simulink model "x5Fish_Run6"  (R2024a)
settings: Solver=VariableStepAuto  StartTime=0.0  StopTime=sim_time  FixedStep=0.0001  RelTol=1e-3
values from neighbouring files (symbols this model uses):
  A = zeros(numSets, 1)    [CurveFitting_Run4.m]    (also in MidlingFish_Run1.m = [A(1:index-1,:);A(index+1:num_search,:)]; MidliningFishOldSkelFunction.m = [A(1:index-1,:);A(index+1:num_search,:)]; calculateSegmentErrors.m = -v1(2))
  B = zeros(numSets, 1)    [CurveFitting_Run4.m]    (also in calculateSegmentErrors.m = v1(1))
  bodlen = fishlen-head    [FishSimParametersFile_Run5.m]
  bsi = NumOfSegs-1    (= 4)    [FishSimParametersFile_Run5.m]
  C = zeros(numSets, 1)    [CurveFitting_Run4.m]    (also in calculateSegmentErrors.m = -(A * startSegment(1) + B * startSegment(2)))
  D = zeros(NumOfSegs)    [FishSimParametersFile_Run5.m]
  Fish_Gain = -[1,1,1,1,1,1,1,1,1,1, 1,  1, 1, 1, 1, 1, 1, 1, 1, 1, 1, 1, 1, 1, 1, 1, 1, 1, 1, 1]    [FishSimParametersFile_Run5.m]
  fish_model_from_head = 59.1375    [FishSimParametersFile_Run5.m]
  head = fishlen*headsize_factor    [FishSimParametersFile_Run5.m]
  head_dense = head_dense*re_ratio    [DensityFinder.m]    (also in FishSimParametersFile_Run5.m = 0.76522755475)
  seglen = bodlen/bsi    [FishSimParametersFile_Run5.m]
  sim_time = t_diff*numel(midlineFiles)    [FishSimParametersFile_Run5.m]
  trunk_dense = trunk_dense*re_ratio    [DensityFinder.m]    (also in FishSimParametersFile_Run5.m = 0.76522755475)
  var_a = fish_width_half_trunk*2*lsf    (= 30.2916666667)    [FishSimParametersFile_Run5.m]
  var_b = var_a- (fish_cross_area_trunk)*(lsf^2)/var_c    (= 6.50064730042)    [FishSimParametersFile_Run5.m]
  var_c = fish_height_half*2*lsf    (= 40.8426966292)    [FishSimParametersFile_Run5.m]
undefined symbols (not defined in the file or in its folder): X, Y, Z
libraries: nesl_utility x63, sm_lib x51
(part 3 of 3)

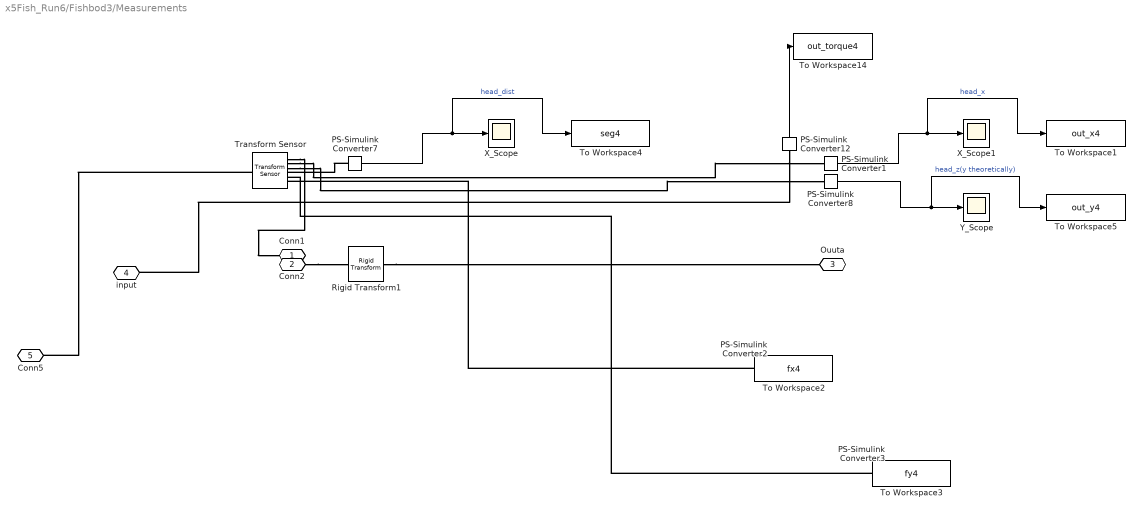
== system x5Fish_Run6/Fishbod3/Measurements ==
  PS-Simulink Converter{1..3,7..8,12} (6 alike) : nesl_utility/PS-Simulink Converter  PhysicalDomain=network_engine_domain  SubClassName=ps_output  LeftPortType=input  RightPortType=output  PseudoPeriodic=off  Frequencies=[]  VectorFormat=inherit  Unit=inherit  AffineConversion=off
  Rigid Transform1 : sm_lib/Frames and Transforms/Rigid Transform  RotationMethod=AlignedAxes  FollAlignAxisA=+Y  BaseAlignAxisA=+Z  FollAlignAxisB=+Z  BaseAlignAxisB=+Y  RotationStandardAxis=+X  RotationAngle=15  RotationAngleUnits=deg  RotationArbitraryAxis=[0 0 1]  RotationSequenceAxes=FollowerAxes  RotationSequence=XYX  RotationSequenceAngles=[0 0 0]  RotationSequenceAnglesUnits=deg  RotationMatrix=[1 0 0; 0 1 0; 0 0 1]  Quaternion=[1 0 0 0]  TranslationMethod=Cartesian  TranslationCartesianOffset=[0.0 0 -(10-5.45)/bsi-2.5]  TranslationCartesianOffsetUnits=mm  TranslationStandardAxis=+Z  TranslationStandardOffset=0  TranslationStandardOffsetUnits=m  TranslationROffset=0  TranslationROffsetUnits=m  TranslationThetaOffset=0  TranslationThetaOffsetUnits=deg  TranslationZOffset=0  TranslationZOffsetUnits=m
  To Workspace1 : ToWorkspace  VariableName=out_x4  SaveFormat=Structure With Time  SampleTime=-1
  To Workspace14 : ToWorkspace  VariableName=out_torque4  SaveFormat=Structure With Time  SampleTime=-1
  To Workspace2 : ToWorkspace  VariableName=fx4  SaveFormat=Structure With Time  SampleTime=-1
  To Workspace3 : ToWorkspace  VariableName=fy4  SaveFormat=Structure With Time  SampleTime=-1
  To Workspace4 : ToWorkspace  VariableName=seg4  SaveFormat=Structure With Time  SampleTime=-1
  To Workspace5 : ToWorkspace  VariableName=out_y4  SaveFormat=Structure With Time  SampleTime=-1
  Transform Sensor : sm_lib/Frames and Transforms/Transform Sensor  MeasurementFrame=World  RotationSequence=XYX  SenseAngle=off  SenseAxis=off  SenseQ=off  SenseR=off  SenseRotationSequence=off  SenseOmegaX=off  SenseOmegaY=off  SenseOmegaZ=off  SenseOmega=off  SenseQDot=off  SenseRDot=off  SenseRotationSequenceDot=off  SenseAlphaX=off  SenseAlphaY=off  SenseAlphaZ=off  SenseAlpha=off  SenseQDDot=off  SenseRDDot=off  SenseX=on  SenseY=on  SenseZ=off  SenseXYZ=off  SenseRad=off  SenseAzim=off  SenseDist=on  SenseInc=off  SenseXDot=off  SenseYDot=off  SenseZDot=off  SenseXYZDot=off  SenseRadDot=off  SenseAzimDot=off  SenseDistDot=off  SenseIncDot=off  SenseXDDot=on  SenseYDDot=on  SenseZDDot=off  SenseXYZDDot=off  SenseRadDDot=off  SenseAzimDDot=off  SenseDistDDot=off  SenseIncDDot=off
  X_Scope : Scope
  X_Scope1 : Scope
  Y_Scope : Scope
  Conn1 : PMIOPort  Side=Right
  Conn2 : PMIOPort  Port=2  Side=Left
  Ouuta : PMIOPort  Port=3  Side=Right
  input : PMIOPort  Port=4  Side=Left
  Conn5 : PMIOPort  Port=5  Side=Left
  wires:
  PS-Simulink Converter8/1 -> To Workspace5/1, Y_Scope/1  "head_z(y theoretically)"
  PS-Simulink Converter1/1 -> To Workspace1/1, X_Scope1/1  "head_x"
  PS-Simulink Converter12/1 -> To Workspace14/1
  PS-Simulink Converter7/1 -> To Workspace4/1, X_Scope/1  "head_dist"
  connections:
  Transform Sensor/RConn2 -- PS-Simulink Converter1/LConn1
  PS-Simulink Converter7/LConn1 -- Transform Sensor/RConn4
  Transform Sensor/RConn3 -- PS-Simulink Converter8/LConn1
  Rigid Transform1/RConn1 -- Ouuta/RConn1
  Transform Sensor/RConn1 -- Conn1/RConn1
  PS-Simulink Converter12/LConn1 -- input/RConn1
  Conn2/RConn1 -- Rigid Transform1/LConn1
  Transform Sensor/LConn1 -- Conn5/RConn1
  PS-Simulink Converter2/LConn1 -- Transform Sensor/RConn6
  PS-Simulink Converter3/LConn1 -- Transform Sensor/RConn5

== system x5Fish_Run6/Fishbod3/Subsystem2 ==
  Mux : Mux  Inputs=2
  To Workspace1 : ToWorkspace  VariableName=f_bot_4  SaveFormat=Structure With Time  SampleTime=-1
  ff_b2 : nesl_utility/PS-Simulink Converter  PhysicalDomain=network_engine_domain  SubClassName=ps_output  LeftPortType=input  RightPortType=output  PseudoPeriodic=off  Frequencies=[]  VectorFormat=inherit  Unit=inherit  AffineConversion=off
  fn_b2 : nesl_utility/PS-Simulink Converter  PhysicalDomain=network_engine_domain  SubClassName=ps_output  LeftPortType=input  RightPortType=output  PseudoPeriodic=off  Frequencies=[]  VectorFormat=inherit  Unit=inherit  AffineConversion=off
  scope contact bot2 : Scope  NumInputPorts=2
  fn : PMIOPort  Side=Left
  ff : PMIOPort  Port=2  Side=Left
  wires:
  ff_b2/1 -> scope contact bot2/2, Mux/2
  fn_b2/1 -> scope contact bot2/1, Mux/1
  Mux/1 -> To Workspace1/1
  connections:
  fn_b2/LConn1 -- fn/RConn1
  ff_b2/LConn1 -- ff/RConn1

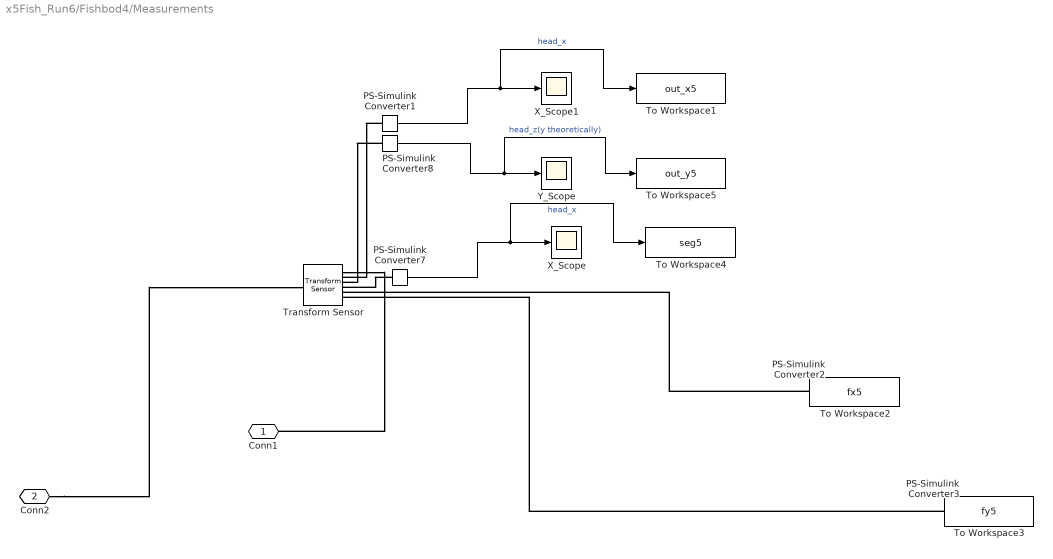
== system x5Fish_Run6/Fishbod4/Measurements ==
  PS-Simulink Converter{1..3,7..8} (5 alike) : nesl_utility/PS-Simulink Converter  PhysicalDomain=network_engine_domain  SubClassName=ps_output  LeftPortType=input  RightPortType=output  PseudoPeriodic=off  Frequencies=[]  VectorFormat=inherit  Unit=inherit  AffineConversion=off
  To Workspace1 : ToWorkspace  VariableName=out_x5  SaveFormat=Structure With Time  SampleTime=-1
  To Workspace2 : ToWorkspace  VariableName=fx5  SaveFormat=Structure With Time  SampleTime=-1
  To Workspace3 : ToWorkspace  VariableName=fy5  SaveFormat=Structure With Time  SampleTime=-1
  To Workspace4 : ToWorkspace  VariableName=seg5  SaveFormat=Structure With Time  SampleTime=-1
  To Workspace5 : ToWorkspace  VariableName=out_y5  SaveFormat=Structure With Time  SampleTime=-1
  Transform Sensor : sm_lib/Frames and Transforms/Transform Sensor  MeasurementFrame=World  RotationSequence=XYX  SenseAngle=off  SenseAxis=off  SenseQ=off  SenseR=off  SenseRotationSequence=off  SenseOmegaX=off  SenseOmegaY=off  SenseOmegaZ=off  SenseOmega=off  SenseQDot=off  SenseRDot=off  SenseRotationSequenceDot=off  SenseAlphaX=off  SenseAlphaY=off  SenseAlphaZ=off  SenseAlpha=off  SenseQDDot=off  SenseRDDot=off  SenseX=on  SenseY=on  SenseZ=off  SenseXYZ=off  SenseRad=off  SenseAzim=off  SenseDist=on  SenseInc=off  SenseXDot=off  SenseYDot=off  SenseZDot=off  SenseXYZDot=off  SenseRadDot=off  SenseAzimDot=off  SenseDistDot=off  SenseIncDot=off  SenseXDDot=on  SenseYDDot=on  SenseZDDot=off  SenseXYZDDot=off  SenseRadDDot=off  SenseAzimDDot=off  SenseDistDDot=off  SenseIncDDot=off
  X_Scope : Scope
  X_Scope1 : Scope
  Y_Scope : Scope
  Conn1 : PMIOPort  Side=Right
  Conn2 : PMIOPort  Port=2  Side=Left
  wires:
  PS-Simulink Converter7/1 -> To Workspace4/1, X_Scope/1  "head_x"
  PS-Simulink Converter8/1 -> To Workspace5/1, Y_Scope/1  "head_z(y theoretically)"
  PS-Simulink Converter1/1 -> To Workspace1/1, X_Scope1/1  "head_x"
  connections:
  Conn2/RConn1 -- Transform Sensor/LConn1
  PS-Simulink Converter8/LConn1 -- Transform Sensor/RConn3
  PS-Simulink Converter1/LConn1 -- Transform Sensor/RConn2
  Transform Sensor/RConn1 -- Conn1/RConn1
  PS-Simulink Converter7/LConn1 -- Transform Sensor/RConn4
  PS-Simulink Converter2/LConn1 -- Transform Sensor/RConn5
  PS-Simulink Converter3/LConn1 -- Transform Sensor/RConn6

== system x5Fish_Run6/Fishbod4/Subsystem2 ==
  Mux : Mux  Inputs=2
  To Workspace1 : ToWorkspace  VariableName=f_bot_5  SaveFormat=Structure With Time  SampleTime=-1
  ff_b2 : nesl_utility/PS-Simulink Converter  PhysicalDomain=network_engine_domain  SubClassName=ps_output  LeftPortType=input  RightPortType=output  PseudoPeriodic=off  Frequencies=[]  VectorFormat=inherit  Unit=inherit  AffineConversion=off
  fn_b2 : nesl_utility/PS-Simulink Converter  PhysicalDomain=network_engine_domain  SubClassName=ps_output  LeftPortType=input  RightPortType=output  PseudoPeriodic=off  Frequencies=[]  VectorFormat=inherit  Unit=inherit  AffineConversion=off
  scope contact bot2 : Scope  NumInputPorts=2
  fn : PMIOPort  Side=Left
  ff : PMIOPort  Port=2  Side=Left
  wires:
  ff_b2/1 -> scope contact bot2/2, Mux/2
  fn_b2/1 -> scope contact bot2/1, Mux/1
  Mux/1 -> To Workspace1/1
  connections:
  fn_b2/LConn1 -- fn/RConn1
  ff_b2/LConn1 -- ff/RConn1
